simulink model "TEP_Final_NoScript"  (R2024a)
settings: Solver=FixedStepAuto  StartTime=0.0  StopTime=10  FixedStep=1/3600  RelTol=1e-3
model workspace (MAT data in the model file):
  AD : Simulink.Parameter (value not decoded)
  AG : Simulink.Parameter (value not decoded)
  AH : Simulink.Parameter (value not decoded)
  AV : Simulink.Parameter (value not decoded)
  AVP : Simulink.Parameter (value not decoded)
  BCHL : Simulink.Parameter (value not decoded)
  BCHV : Simulink.Parameter (value not decoded)
  BD : Simulink.Parameter (value not decoded)
  BG : Simulink.Parameter (value not decoded)
  BH : Simulink.Parameter (value not decoded)
  BVP : Simulink.Parameter (value not decoded)
  CD : Simulink.Parameter (value not decoded)
  CG : Simulink.Parameter (value not decoded)
  CH : Simulink.Parameter (value not decoded)
  CVP : Simulink.Parameter (value not decoded)
  XMW : Simulink.Parameter (value not decoded)
  XNS : Simulink.Parameter (value not decoded)
  XNSE : Simulink.Parameter (value not decoded)
symbols that are objects in the model workspace (value not decoded): AD, AG, AH, AV, AVP, BD, BG, BH, BVP, CD, CG, CH, CVP, XMW, XNS, XNSE
undefined symbols (not defined in the file or in its folder): magnitude, msgbox, SETPT, XMEAS, XMV
libraries: mylib x360, dspindex x28
(part 12 of 14)

== system TEP_Final_NoScript/Subsystem1/RCout/Subsystem3/Subsystem/Subsystem2 ==
  T1 : Inport
  T0 : Inport  Port=2
  A : Constant  Value=9.069
  Add1 : Sum  Inputs=+-
  Product1 : Product
  AT : Outport
  wires:
  Add1/1 -> Product1/2
  A/1 -> Product1/1
  T0/1 -> Add1/2
  T1/1 -> Add1/1
  Product1/1 -> AT/1

== system TEP_Final_NoScript/Subsystem1/RCout/Subsystem3/Subsystem1/Subsystem ==
  T1 : Inport
  T0 : Inport  Port=2
  A : Constant  Value=9.069
  Divide : Product  Inputs=*/
  Math Function : Math  Operator=log  SignedPower=on
  Product1 : Product
  AT : Outport
  wires:
  Product1/1 -> AT/1
  A/1 -> Product1/1
  T1/1 -> Divide/1
  T0/1 -> Divide/2
  Math Function/1 -> Product1/2
  Divide/1 -> Math Function/1

== system TEP_Final_NoScript/Subsystem1/Reactor feed stream/Composition measurement mol%/Subsystem/Subsystem ==
  XST : Inport
  Constant : Constant  Value=100
  Multiport Selector : dspindex/Multiport Selector  rowsOrCols=Rows  idxCellArray={7,8}  idxErrMode=Clip Index
  Product6 : Product
  Product7 : Product
  XCMPG : Outport  VectorParamsAs1DForOutWhenUnconnected=off
  "XCMPH " : Outport  Port=2  VectorParamsAs1DForOutWhenUnconnected=off
  wires:
  Multiport Selector/2 -> Product7/1
  Multiport Selector/1 -> Product6/1
  Constant/1 -> Product6/2, Product7/2
  XST/1 -> Multiport Selector/1
  Product6/1 -> XCMPG/1
  Product7/1 -> "XCMPH "/1

== system TEP_Final_NoScript/Subsystem1/Reactor product stream/Composition measurement mol%/Subsystem/Subsystem ==
  XST : Inport
  Constant : Constant  Value=100
  Multiport Selector : dspindex/Multiport Selector  rowsOrCols=Rows  idxCellArray={ 1,2,3,4,5,6,7,8}  idxErrMode=Clip Index
  Product{,1..7} (8 alike) : Product
  XCMPA : Outport  VectorParamsAs1DForOutWhenUnconnected=off
  XCMPB : Outport  Port=2  VectorParamsAs1DForOutWhenUnconnected=off
  XCMPC : Outport  Port=3  VectorParamsAs1DForOutWhenUnconnected=off
  XCMPD : Outport  Port=4  VectorParamsAs1DForOutWhenUnconnected=off
  "XCMPE " : Outport  Port=5  VectorParamsAs1DForOutWhenUnconnected=off
  "XCMPF " : Outport  Port=6  VectorParamsAs1DForOutWhenUnconnected=off
  XCMPG : Outport  Port=7  VectorParamsAs1DForOutWhenUnconnected=off
  "XCMPH " : Outport  Port=8  VectorParamsAs1DForOutWhenUnconnected=off
  wires:
  Multiport Selector/6 -> Product5/1
  Multiport Selector/8 -> Product7/1
  Multiport Selector/5 -> Product4/1
  Multiport Selector/7 -> Product6/1
  Multiport Selector/1 -> Product/1
  Multiport Selector/3 -> Product2/1
  Constant/1 -> Product/2, Product1/2, Product2/2, Product3/2, Product4/2, Product5/2, Product7/2, Product6/2
  Multiport Selector/4 -> Product3/1
  XST/1 -> Multiport Selector/1
  Multiport Selector/2 -> Product1/1
  Product/1 -> XCMPA/1
  Product1/1 -> XCMPB/1
  Product2/1 -> XCMPC/1
  Product3/1 -> XCMPD/1
  Product4/1 -> "XCMPE "/1
  Product5/1 -> "XCMPF "/1
  Product6/1 -> XCMPG/1
  Product7/1 -> "XCMPH "/1

== system TEP_Final_NoScript/Subsystem1/Separator recycle stream/Composition measurement mol%/Subsystem/Subsystem ==
  XST : Inport
  Constant : Constant  Value=100
  Multiport Selector : dspindex/Multiport Selector  rowsOrCols=Rows  idxCellArray={ 1,2,3,4,5,6,7,8}  idxErrMode=Clip Index
  Product{,1..7} (8 alike) : Product
  XCMPA : Outport  VectorParamsAs1DForOutWhenUnconnected=off
  XCMPB : Outport  Port=2  VectorParamsAs1DForOutWhenUnconnected=off
  XCMPC : Outport  Port=3  VectorParamsAs1DForOutWhenUnconnected=off
  XCMPD : Outport  Port=4  VectorParamsAs1DForOutWhenUnconnected=off
  "XCMPE " : Outport  Port=5  VectorParamsAs1DForOutWhenUnconnected=off
  "XCMPF " : Outport  Port=6  VectorParamsAs1DForOutWhenUnconnected=off
  XCMPG : Outport  Port=7  VectorParamsAs1DForOutWhenUnconnected=off
  "XCMPH " : Outport  Port=8  VectorParamsAs1DForOutWhenUnconnected=off
  wires:
  Multiport Selector/6 -> Product5/1
  Multiport Selector/8 -> Product7/1
  Multiport Selector/5 -> Product4/1
  Multiport Selector/7 -> Product6/1
  Multiport Selector/1 -> Product/1
  Multiport Selector/3 -> Product2/1
  Constant/1 -> Product/2, Product1/2, Product2/2, Product3/2, Product4/2, Product5/2, Product7/2, Product6/2
  Multiport Selector/4 -> Product3/1
  XST/1 -> Multiport Selector/1
  Multiport Selector/2 -> Product1/1
  Product/1 -> XCMPA/1
  Product1/1 -> XCMPB/1
  Product2/1 -> XCMPC/1
  Product3/1 -> XCMPD/1
  Product4/1 -> "XCMPE "/1
  Product5/1 -> "XCMPF "/1
  Product6/1 -> XCMPG/1
  Product7/1 -> "XCMPH "/1

== system TEP_Final_NoScript/Subsystem1/Separator underflow stream/Composition measurement mol%/Subsystem/Subsystem ==
  XST : Inport
  Constant : Constant  Value=100
  Multiport Selector : dspindex/Multiport Selector  rowsOrCols=Rows  idxCellArray={ 1,2,3,4,5,6,7,8}  idxErrMode=Clip Index
  Product{,1..7} (8 alike) : Product
  XCMPA : Outport  VectorParamsAs1DForOutWhenUnconnected=off
  XCMPB : Outport  Port=2  VectorParamsAs1DForOutWhenUnconnected=off
  XCMPC : Outport  Port=3  VectorParamsAs1DForOutWhenUnconnected=off
  XCMPD : Outport  Port=4  VectorParamsAs1DForOutWhenUnconnected=off
  "XCMPE " : Outport  Port=5  VectorParamsAs1DForOutWhenUnconnected=off
  "XCMPF " : Outport  Port=6  VectorParamsAs1DForOutWhenUnconnected=off
  XCMPG : Outport  Port=7  VectorParamsAs1DForOutWhenUnconnected=off
  "XCMPH " : Outport  Port=8  VectorParamsAs1DForOutWhenUnconnected=off
  wires:
  Multiport Selector/6 -> Product5/1
  Multiport Selector/8 -> Product7/1
  Multiport Selector/5 -> Product4/1
  Multiport Selector/7 -> Product6/1
  Multiport Selector/1 -> Product/1
  Multiport Selector/3 -> Product2/1
  Constant/1 -> Product/2, Product1/2, Product2/2, Product3/2, Product4/2, Product5/2, Product7/2, Product6/2
  Multiport Selector/4 -> Product3/1
  XST/1 -> Multiport Selector/1
  Multiport Selector/2 -> Product1/1
  Product/1 -> XCMPA/1
  Product1/1 -> XCMPB/1
  Product2/1 -> XCMPC/1
  Product3/1 -> XCMPD/1
  Product4/1 -> "XCMPE "/1
  Product5/1 -> "XCMPF "/1
  Product6/1 -> XCMPG/1
  Product7/1 -> "XCMPH "/1

== system TEP_Final_NoScript/Subsystem1/Stripper recycle stream/Composition measurement mol%/Subsystem/Subsystem ==
  XST : Inport
  Constant : Constant  Value=100
  Multiport Selector : dspindex/Multiport Selector  rowsOrCols=Rows  idxCellArray={ 1,2,3,4,5,6,7,8}  idxErrMode=Clip Index
  Product{,1..7} (8 alike) : Product
  XCMPA : Outport  VectorParamsAs1DForOutWhenUnconnected=off
  XCMPB : Outport  Port=2  VectorParamsAs1DForOutWhenUnconnected=off
  XCMPC : Outport  Port=3  VectorParamsAs1DForOutWhenUnconnected=off
  XCMPD : Outport  Port=4  VectorParamsAs1DForOutWhenUnconnected=off
  "XCMPE " : Outport  Port=5  VectorParamsAs1DForOutWhenUnconnected=off
  "XCMPF " : Outport  Port=6  VectorParamsAs1DForOutWhenUnconnected=off
  XCMPG : Outport  Port=7  VectorParamsAs1DForOutWhenUnconnected=off
  "XCMPH " : Outport  Port=8  VectorParamsAs1DForOutWhenUnconnected=off
  wires:
  Multiport Selector/6 -> Product5/1
  Multiport Selector/8 -> Product7/1
  Multiport Selector/5 -> Product4/1
  Multiport Selector/7 -> Product6/1
  Multiport Selector/1 -> Product/1
  Multiport Selector/3 -> Product2/1
  Constant/1 -> Product/2, Product1/2, Product2/2, Product3/2, Product4/2, Product5/2, Product7/2, Product6/2
  Multiport Selector/4 -> Product3/1
  XST/1 -> Multiport Selector/1
  Multiport Selector/2 -> Product1/1
  Product/1 -> XCMPA/1
  Product1/1 -> XCMPB/1
  Product2/1 -> XCMPC/1
  Product3/1 -> XCMPD/1
  Product4/1 -> "XCMPE "/1
  Product5/1 -> "XCMPF "/1
  Product6/1 -> XCMPG/1
  Product7/1 -> "XCMPH "/1

== system TEP_Final_NoScript/Subsystem1/Subsystem1/Subsystem1/Flow measurement in lb-mol//hr/XMWS Molecular weight of Stream lb//lb-mol ==
  XST : Inport
  Product : Product
  Sum of Elements : Sum  Inputs=+
  "XMW(I) Molecular weight of components lb/lb-mol " : Constant  Value=XMW
  XMWS : Outport  VectorParamsAs1DForOutWhenUnconnected=off
  wires:
  Sum of Elements/1 -> XMWS/1
  Product/1 -> Sum of Elements/1
  XST/1 -> Product/1
  "XMW(I) Molecular weight of components lb/lb-mol "/1 -> Product/2

== system TEP_Final_NoScript/Subsystem1/Subsystem13/Subsystem1/Flow measurement in lb-mol//hr/XMWS Molecular weight of Stream lb//lb-mol ==
  XST : Inport
  Product : Product
  Sum of Elements : Sum  Inputs=+
  "XMW(I) Molecular weight of components lb/lb-mol " : Constant  Value=XMW
  XMWS : Outport  VectorParamsAs1DForOutWhenUnconnected=off
  wires:
  Sum of Elements/1 -> XMWS/1
  Product/1 -> Sum of Elements/1
  XST/1 -> Product/1
  "XMW(I) Molecular weight of components lb/lb-mol "/1 -> Product/2

== system TEP_Final_NoScript/Subsystem1/Subsystem14/Subsystem1/Flow measurement in lb-mol//hr/XMWS Molecular weight of Stream lb//lb-mol ==
  XST : Inport
  Product : Product
  Sum of Elements : Sum  Inputs=+
  "XMW(I) Molecular weight of components lb/lb-mol " : Constant  Value=XMW
  XMWS : Outport  VectorParamsAs1DForOutWhenUnconnected=off
  wires:
  Sum of Elements/1 -> XMWS/1
  Product/1 -> Sum of Elements/1
  XST/1 -> Product/1
  "XMW(I) Molecular weight of components lb/lb-mol "/1 -> Product/2

== system TEP_Final_NoScript/Subsystem1/Subsystem15/Subsystem1/Flow measurement in lb-mol//hr/XMWS Molecular weight of Stream lb//lb-mol ==
  XST : Inport
  Product : Product
  Sum of Elements : Sum  Inputs=+
  "XMW(I) Molecular weight of components lb/lb-mol " : Constant  Value=XMW
  XMWS : Outport  VectorParamsAs1DForOutWhenUnconnected=off
  wires:
  Sum of Elements/1 -> XMWS/1
  Product/1 -> Sum of Elements/1
  XST/1 -> Product/1
  "XMW(I) Molecular weight of components lb/lb-mol "/1 -> Product/2

== system TEP_Final_NoScript/Subsystem1/Subsystem16/Subsystem1/Flow measurement in lb-mol//hr/XMWS Molecular weight of Stream lb//lb-mol ==
  XST : Inport
  Product : Product
  Sum of Elements : Sum  Inputs=+
  "XMW(I) Molecular weight of components lb/lb-mol " : Constant  Value=XMW
  XMWS : Outport  VectorParamsAs1DForOutWhenUnconnected=off
  wires:
  Sum of Elements/1 -> XMWS/1
  Product/1 -> Sum of Elements/1
  XST/1 -> Product/1
  "XMW(I) Molecular weight of components lb/lb-mol "/1 -> Product/2

== system TEP_Final_NoScript/Subsystem1/Subsystem17/Subsystem1/Flow measurement in lb-mol//hr/XMWS Molecular weight of Stream lb//lb-mol ==
  XST : Inport
  Product : Product
  Sum of Elements : Sum  Inputs=+
  "XMW(I) Molecular weight of components lb/lb-mol " : Constant  Value=XMW
  XMWS : Outport  VectorParamsAs1DForOutWhenUnconnected=off
  wires:
  Sum of Elements/1 -> XMWS/1
  Product/1 -> Sum of Elements/1
  XST/1 -> Product/1
  "XMW(I) Molecular weight of components lb/lb-mol "/1 -> Product/2

== system TEP_Final_NoScript/Subsystem1/Subsystem2/Subsystem1/Flow measurement in lb-mol//hr/XMWS Molecular weight of Stream lb//lb-mol ==
  XST : Inport
  Product : Product
  Sum of Elements : Sum  Inputs=+
  "XMW(I) Molecular weight of components lb/lb-mol " : Constant  Value=XMW
  XMWS : Outport  VectorParamsAs1DForOutWhenUnconnected=off
  wires:
  Sum of Elements/1 -> XMWS/1
  Product/1 -> Sum of Elements/1
  XST/1 -> Product/1
  "XMW(I) Molecular weight of components lb/lb-mol "/1 -> Product/2

== system TEP_Final_NoScript/Subsystem1/Subsystem3/Subsystem1/Flow measurement in lb-mol//hr/XMWS Molecular weight of Stream lb//lb-mol ==
  XST : Inport
  Product : Product
  Sum of Elements : Sum  Inputs=+
  "XMW(I) Molecular weight of components lb/lb-mol " : Constant  Value=XMW
  XMWS : Outport  VectorParamsAs1DForOutWhenUnconnected=off
  wires:
  Sum of Elements/1 -> XMWS/1
  Product/1 -> Sum of Elements/1
  XST/1 -> Product/1
  "XMW(I) Molecular weight of components lb/lb-mol "/1 -> Product/2

== system TEP_Final_NoScript/Subsystem1/Subsystem4/Subsystem1/Flow measurement in lb-mol//hr/XMWS Molecular weight of Stream lb//lb-mol ==
  XST : Inport
  Product : Product
  Sum of Elements : Sum  Inputs=+
  "XMW(I) Molecular weight of components lb/lb-mol " : Constant  Value=XMW
  XMWS : Outport  VectorParamsAs1DForOutWhenUnconnected=off
  wires:
  Sum of Elements/1 -> XMWS/1
  Product/1 -> Sum of Elements/1
  XST/1 -> Product/1
  "XMW(I) Molecular weight of components lb/lb-mol "/1 -> Product/2

== system TEP_Final_NoScript/Subsystem1/Subsystem5/Subsystem1/Flow measurement in lb-mol//hr/XMWS Molecular weight of Stream lb//lb-mol ==
  XST : Inport
  Product : Product
  Sum of Elements : Sum  Inputs=+
  "XMW(I) Molecular weight of components lb/lb-mol " : Constant  Value=XMW
  XMWS : Outport  VectorParamsAs1DForOutWhenUnconnected=off
  wires:
  Sum of Elements/1 -> XMWS/1
  Product/1 -> Sum of Elements/1
  XST/1 -> Product/1
  "XMW(I) Molecular weight of components lb/lb-mol "/1 -> Product/2

== system TEP_Final_NoScript/Subsystem1/Subsystem8/Subsystem1/Flow measurement in lb-mol//hr/XMWS Molecular weight of Stream lb//lb-mol ==
  XST : Inport
  Product : Product
  Sum of Elements : Sum  Inputs=+
  "XMW(I) Molecular weight of components lb/lb-mol " : Constant  Value=XMW
  XMWS : Outport  VectorParamsAs1DForOutWhenUnconnected=off
  wires:
  Sum of Elements/1 -> XMWS/1
  Product/1 -> Sum of Elements/1
  XST/1 -> Product/1
  "XMW(I) Molecular weight of components lb/lb-mol "/1 -> Product/2

== system TEP_Final_NoScript/Random number generator1/Process Measurements XMEAS(I) I=23-36/If Action Subsystem3/Subsystem/Subsystem/TESUB6 XMNS(23) ==
  G : Inport
  Process Noise I=1-12 G New : mylib/Process Noise I=1-12 G New  SystemSampleTime=-1  VariantActivationTime=update diagram  AllowFlexibleInterface=on  Latency=0  AutoFrameSizeCalculation=off
      settings: SourceProductName=TEP Library
  XNS(23) : Constant  Value=0.25
  XMNS : Outport  VectorParamsAs1DForOutWhenUnconnected=off
  G_NEW : Outport  Port=2  VectorParamsAs1DForOutWhenUnconnected=off
  wires:
  XNS(23)/1 -> Process Noise I=1-12 G New/1
  Process Noise I=1-12 G New/1 -> XMNS/1
  G/1 -> Process Noise I=1-12 G New/2
  Process Noise I=1-12 G New/2 -> G_NEW/1

== system TEP_Final_NoScript/Random number generator1/Process Measurements XMEAS(I) I=23-36/If Action Subsystem3/Subsystem/Subsystem/TESUB6 XMNS(24) ==
  G : Inport
  Process Noise I=1-12 G New : mylib/Process Noise I=1-12 G New  SystemSampleTime=-1  VariantActivationTime=update diagram  AllowFlexibleInterface=on  Latency=0  AutoFrameSizeCalculation=off
      settings: SourceProductName=TEP Library
  XNS(24) : Constant  Value=0.1
  XMNS : Outport  VectorParamsAs1DForOutWhenUnconnected=off
  G_NEW : Outport  Port=2  VectorParamsAs1DForOutWhenUnconnected=off
  wires:
  XNS(24)/1 -> Process Noise I=1-12 G New/1
  Process Noise I=1-12 G New/1 -> XMNS/1
  G/1 -> Process Noise I=1-12 G New/2
  Process Noise I=1-12 G New/2 -> G_NEW/1

== system TEP_Final_NoScript/Random number generator1/Process Measurements XMEAS(I) I=23-36/If Action Subsystem3/Subsystem/Subsystem/TESUB6 XMNS(25) ==
  G : Inport
  Process Noise I=1-12 G New : mylib/Process Noise I=1-12 G New  SystemSampleTime=-1  VariantActivationTime=update diagram  AllowFlexibleInterface=on  Latency=0  AutoFrameSizeCalculation=off
      settings: SourceProductName=TEP Library
  XNS(25) : Constant  Value=0.25
  XMNS : Outport  VectorParamsAs1DForOutWhenUnconnected=off
  G_NEW : Outport  Port=2  VectorParamsAs1DForOutWhenUnconnected=off
  wires:
  XNS(25)/1 -> Process Noise I=1-12 G New/1
  Process Noise I=1-12 G New/1 -> XMNS/1
  G/1 -> Process Noise I=1-12 G New/2
  Process Noise I=1-12 G New/2 -> G_NEW/1

== system TEP_Final_NoScript/Random number generator1/Process Measurements XMEAS(I) I=23-36/If Action Subsystem3/Subsystem/Subsystem/TESUB6 XMNS(26) ==
  G : Inport
  Process Noise I=1-12 G New : mylib/Process Noise I=1-12 G New  SystemSampleTime=-1  VariantActivationTime=update diagram  AllowFlexibleInterface=on  Latency=0  AutoFrameSizeCalculation=off
      settings: SourceProductName=TEP Library
  XNS(26) : Constant  Value=0.1
  XMNS : Outport  VectorParamsAs1DForOutWhenUnconnected=off
  G_NEW : Outport  Port=2  VectorParamsAs1DForOutWhenUnconnected=off
  wires:
  XNS(26)/1 -> Process Noise I=1-12 G New/1
  Process Noise I=1-12 G New/1 -> XMNS/1
  G/1 -> Process Noise I=1-12 G New/2
  Process Noise I=1-12 G New/2 -> G_NEW/1

== system TEP_Final_NoScript/Random number generator1/Process Measurements XMEAS(I) I=23-36/If Action Subsystem3/Subsystem/Subsystem/TESUB6 XMNS(27) ==
  G : Inport
  Process Noise I=1-12 G New : mylib/Process Noise I=1-12 G New  SystemSampleTime=-1  VariantActivationTime=update diagram  AllowFlexibleInterface=on  Latency=0  AutoFrameSizeCalculation=off
      settings: SourceProductName=TEP Library
  XNS(27) : Constant  Value=0.25
  XMNS : Outport  VectorParamsAs1DForOutWhenUnconnected=off
  G_NEW : Outport  Port=2  VectorParamsAs1DForOutWhenUnconnected=off
  wires:
  XNS(27)/1 -> Process Noise I=1-12 G New/1
  Process Noise I=1-12 G New/1 -> XMNS/1
  G/1 -> Process Noise I=1-12 G New/2
  Process Noise I=1-12 G New/2 -> G_NEW/1

== system TEP_Final_NoScript/Random number generator1/Process Measurements XMEAS(I) I=23-36/If Action Subsystem3/Subsystem/Subsystem1/TESUB6 XMNS(28) ==
  G : Inport
  Process Noise I=1-12 G New : mylib/Process Noise I=1-12 G New  SystemSampleTime=-1  VariantActivationTime=update diagram  AllowFlexibleInterface=on  Latency=0  AutoFrameSizeCalculation=off
      settings: SourceProductName=TEP Library
  XNS(28) : Constant  Value=0.025
  XMNS : Outport  VectorParamsAs1DForOutWhenUnconnected=off
  G_NEW : Outport  Port=2  VectorParamsAs1DForOutWhenUnconnected=off
  wires:
  XNS(28)/1 -> Process Noise I=1-12 G New/1
  Process Noise I=1-12 G New/1 -> XMNS/1
  G/1 -> Process Noise I=1-12 G New/2
  Process Noise I=1-12 G New/2 -> G_NEW/1

== system TEP_Final_NoScript/Random number generator1/Process Measurements XMEAS(I) I=23-36/If Action Subsystem3/Subsystem/Subsystem1/TESUB6 XMNS(29) ==
  G : Inport
  Process Noise I=1-12 G New : mylib/Process Noise I=1-12 G New  SystemSampleTime=-1  VariantActivationTime=update diagram  AllowFlexibleInterface=on  Latency=0  AutoFrameSizeCalculation=off
      settings: SourceProductName=TEP Library
  XNS(29) : Constant  Value=0.25
  XMNS : Outport  VectorParamsAs1DForOutWhenUnconnected=off
  G_NEW : Outport  Port=2  VectorParamsAs1DForOutWhenUnconnected=off
  wires:
  XNS(29)/1 -> Process Noise I=1-12 G New/1
  Process Noise I=1-12 G New/1 -> XMNS/1
  G/1 -> Process Noise I=1-12 G New/2
  Process Noise I=1-12 G New/2 -> G_NEW/1

== system TEP_Final_NoScript/Random number generator1/Process Measurements XMEAS(I) I=23-36/If Action Subsystem3/Subsystem/Subsystem1/TESUB6 XMNS(30) ==
  G : Inport
  Process Noise I=1-12 G New : mylib/Process Noise I=1-12 G New  SystemSampleTime=-1  VariantActivationTime=update diagram  AllowFlexibleInterface=on  Latency=0  AutoFrameSizeCalculation=off
      settings: SourceProductName=TEP Library
  XNS(30) : Constant  Value=0.1
  XMNS : Outport  VectorParamsAs1DForOutWhenUnconnected=off
  G_NEW : Outport  Port=2  VectorParamsAs1DForOutWhenUnconnected=off
  wires:
  XNS(30)/1 -> Process Noise I=1-12 G New/1
  Process Noise I=1-12 G New/1 -> XMNS/1
  G/1 -> Process Noise I=1-12 G New/2
  Process Noise I=1-12 G New/2 -> G_NEW/1

== system TEP_Final_NoScript/Random number generator1/Process Measurements XMEAS(I) I=23-36/If Action Subsystem3/Subsystem/Subsystem1/TESUB6 XMNS(31) ==
  G : Inport
  Process Noise I=1-12 G New : mylib/Process Noise I=1-12 G New  SystemSampleTime=-1  VariantActivationTime=update diagram  AllowFlexibleInterface=on  Latency=0  AutoFrameSizeCalculation=off
      settings: SourceProductName=TEP Library
  XNS(31) : Constant  Value=0.25
  XMNS : Outport  VectorParamsAs1DForOutWhenUnconnected=off
  G_NEW : Outport  Port=2  VectorParamsAs1DForOutWhenUnconnected=off
  wires:
  XNS(31)/1 -> Process Noise I=1-12 G New/1
  Process Noise I=1-12 G New/1 -> XMNS/1
  G/1 -> Process Noise I=1-12 G New/2
  Process Noise I=1-12 G New/2 -> G_NEW/1

== system TEP_Final_NoScript/Random number generator1/Process Measurements XMEAS(I) I=23-36/If Action Subsystem3/Subsystem/Subsystem1/TESUB6 XMNS(32) ==
  G : Inport
  Process Noise I=1-12 G New : mylib/Process Noise I=1-12 G New  SystemSampleTime=-1  VariantActivationTime=update diagram  AllowFlexibleInterface=on  Latency=0  AutoFrameSizeCalculation=off
      settings: SourceProductName=TEP Library
  XNS(32) : Constant  Value=0.1
  XMNS : Outport  VectorParamsAs1DForOutWhenUnconnected=off
  G_NEW : Outport  Port=2  VectorParamsAs1DForOutWhenUnconnected=off
  wires:
  XNS(32)/1 -> Process Noise I=1-12 G New/1
  Process Noise I=1-12 G New/1 -> XMNS/1
  G/1 -> Process Noise I=1-12 G New/2
  Process Noise I=1-12 G New/2 -> G_NEW/1

== system TEP_Final_NoScript/Random number generator1/Process Measurements XMEAS(I) I=23-36/If Action Subsystem3/Subsystem/Subsystem2/TESUB6 XMNS(33) ==
  G : Inport
  Process Noise I=1-12 G New : mylib/Process Noise I=1-12 G New  SystemSampleTime=-1  VariantActivationTime=update diagram  AllowFlexibleInterface=on  Latency=0  AutoFrameSizeCalculation=off
      settings: SourceProductName=TEP Library
  XNS(33) : Constant  Value=0.25
  XMNS : Outport  VectorParamsAs1DForOutWhenUnconnected=off
  G_NEW : Outport  Port=2  VectorParamsAs1DForOutWhenUnconnected=off
  wires:
  XNS(33)/1 -> Process Noise I=1-12 G New/1
  Process Noise I=1-12 G New/1 -> XMNS/1
  G/1 -> Process Noise I=1-12 G New/2
  Process Noise I=1-12 G New/2 -> G_NEW/1

== system TEP_Final_NoScript/Random number generator1/Process Measurements XMEAS(I) I=23-36/If Action Subsystem3/Subsystem/Subsystem2/TESUB6 XMNS(34) ==
  G : Inport
  Process Noise I=1-12 G New : mylib/Process Noise I=1-12 G New  SystemSampleTime=-1  VariantActivationTime=update diagram  AllowFlexibleInterface=on  Latency=0  AutoFrameSizeCalculation=off
      settings: SourceProductName=TEP Library
  XNS(34) : Constant  Value=0.025
  XMNS : Outport  VectorParamsAs1DForOutWhenUnconnected=off
  G_NEW : Outport  Port=2  VectorParamsAs1DForOutWhenUnconnected=off
  wires:
  XNS(34)/1 -> Process Noise I=1-12 G New/1
  Process Noise I=1-12 G New/1 -> XMNS/1
  G/1 -> Process Noise I=1-12 G New/2
  Process Noise I=1-12 G New/2 -> G_NEW/1

== system TEP_Final_NoScript/Random number generator1/Process Measurements XMEAS(I) I=23-36/If Action Subsystem3/Subsystem/Subsystem2/TESUB6 XMNS(35) ==
  G : Inport
  Process Noise I=1-12 G New : mylib/Process Noise I=1-12 G New  SystemSampleTime=-1  VariantActivationTime=update diagram  AllowFlexibleInterface=on  Latency=0  AutoFrameSizeCalculation=off
      settings: SourceProductName=TEP Library
  XNS(35) : Constant  Value=0.05
  XMNS : Outport  VectorParamsAs1DForOutWhenUnconnected=off
  G_NEW : Outport  Port=2  VectorParamsAs1DForOutWhenUnconnected=off
  wires:
  XNS(35)/1 -> Process Noise I=1-12 G New/1
  Process Noise I=1-12 G New/1 -> XMNS/1
  G/1 -> Process Noise I=1-12 G New/2
  Process Noise I=1-12 G New/2 -> G_NEW/1

== system TEP_Final_NoScript/Random number generator1/Process Measurements XMEAS(I) I=23-36/If Action Subsystem3/Subsystem/Subsystem2/TESUB6 XMNS(36) ==
  G : Inport
  Process Noise I=1-12 G New : mylib/Process Noise I=1-12 G New  SystemSampleTime=-1  VariantActivationTime=update diagram  AllowFlexibleInterface=on  Latency=0  AutoFrameSizeCalculation=off
      settings: SourceProductName=TEP Library
  XNS(36) : Constant  Value=0.05
  XMNS : Outport  VectorParamsAs1DForOutWhenUnconnected=off
  G_NEW : Outport  Port=2  VectorParamsAs1DForOutWhenUnconnected=off
  wires:
  XNS(36)/1 -> Process Noise I=1-12 G New/1
  Process Noise I=1-12 G New/1 -> XMNS/1
  G/1 -> Process Noise I=1-12 G New/2
  Process Noise I=1-12 G New/2 -> G_NEW/1

== system TEP_Final_NoScript/Random number generator1/Process Measurements XMEAS(I) I=37-41/If Action Subsystem3/Subsystem/Subsystem/TESUB6 XMNS(37) ==
  G : Inport
  Process Noise I=1-12 G New : mylib/Process Noise I=1-12 G New  SystemSampleTime=-1  VariantActivationTime=update diagram  AllowFlexibleInterface=on  Latency=0  AutoFrameSizeCalculation=off
      settings: SourceProductName=TEP Library
  XNS(37) : Constant  Value=0.01
  XMNS : Outport  VectorParamsAs1DForOutWhenUnconnected=off
  G_NEW : Outport  Port=2  VectorParamsAs1DForOutWhenUnconnected=off
  wires:
  XNS(37)/1 -> Process Noise I=1-12 G New/1
  Process Noise I=1-12 G New/1 -> XMNS/1
  G/1 -> Process Noise I=1-12 G New/2
  Process Noise I=1-12 G New/2 -> G_NEW/1

== system TEP_Final_NoScript/Random number generator1/Process Measurements XMEAS(I) I=37-41/If Action Subsystem3/Subsystem/Subsystem/TESUB6 XMNS(38) ==
  G : Inport
  Process Noise I=1-12 G New : mylib/Process Noise I=1-12 G New  SystemSampleTime=-1  VariantActivationTime=update diagram  AllowFlexibleInterface=on  Latency=0  AutoFrameSizeCalculation=off
      settings: SourceProductName=TEP Library
  XNS(38) : Constant  Value=0.01
  XMNS : Outport  VectorParamsAs1DForOutWhenUnconnected=off
  G_NEW : Outport  Port=2  VectorParamsAs1DForOutWhenUnconnected=off
  wires:
  XNS(38)/1 -> Process Noise I=1-12 G New/1
  Process Noise I=1-12 G New/1 -> XMNS/1
  G/1 -> Process Noise I=1-12 G New/2
  Process Noise I=1-12 G New/2 -> G_NEW/1

== system TEP_Final_NoScript/Random number generator1/Process Measurements XMEAS(I) I=37-41/If Action Subsystem3/Subsystem/Subsystem/TESUB6 XMNS(39) ==
  G : Inport
  Process Noise I=1-12 G New : mylib/Process Noise I=1-12 G New  SystemSampleTime=-1  VariantActivationTime=update diagram  AllowFlexibleInterface=on  Latency=0  AutoFrameSizeCalculation=off
      settings: SourceProductName=TEP Library
  XNS(39) : Constant  Value=0.01
  XMNS : Outport  VectorParamsAs1DForOutWhenUnconnected=off
  G_NEW : Outport  Port=2  VectorParamsAs1DForOutWhenUnconnected=off
  wires:
  XNS(39)/1 -> Process Noise I=1-12 G New/1
  Process Noise I=1-12 G New/1 -> XMNS/1
  G/1 -> Process Noise I=1-12 G New/2
  Process Noise I=1-12 G New/2 -> G_NEW/1

== system TEP_Final_NoScript/Random number generator1/Process Measurements XMEAS(I) I=37-41/If Action Subsystem3/Subsystem/Subsystem/TESUB6 XMNS(40) ==
  G : Inport
  Process Noise I=1-12 G New : mylib/Process Noise I=1-12 G New  SystemSampleTime=-1  VariantActivationTime=update diagram  AllowFlexibleInterface=on  Latency=0  AutoFrameSizeCalculation=off
      settings: SourceProductName=TEP Library
  XNS(40) : Constant  Value=0.5
  XMNS : Outport  VectorParamsAs1DForOutWhenUnconnected=off
  G_NEW : Outport  Port=2  VectorParamsAs1DForOutWhenUnconnected=off
  wires:
  XNS(40)/1 -> Process Noise I=1-12 G New/1
  Process Noise I=1-12 G New/1 -> XMNS/1
  G/1 -> Process Noise I=1-12 G New/2
  Process Noise I=1-12 G New/2 -> G_NEW/1

== system TEP_Final_NoScript/Random number generator1/Process Measurements XMEAS(I) I=37-41/If Action Subsystem3/Subsystem/Subsystem/TESUB6 XMNS(41) ==
  G : Inport
  Process Noise I=1-12 G New : mylib/Process Noise I=1-12 G New  SystemSampleTime=-1  VariantActivationTime=update diagram  AllowFlexibleInterface=on  Latency=0  AutoFrameSizeCalculation=off
      settings: SourceProductName=TEP Library
  XNS(41) : Constant  Value=0.5
  XMNS : Outport  VectorParamsAs1DForOutWhenUnconnected=off
  G_NEW : Outport  Port=2  VectorParamsAs1DForOutWhenUnconnected=off
  wires:
  XNS(41)/1 -> Process Noise I=1-12 G New/1
  Process Noise I=1-12 G New/1 -> XMNS/1
  G/1 -> Process Noise I=1-12 G New/2
  Process Noise I=1-12 G New/2 -> G_NEW/1

== system TEP_Final_NoScript/Random number generator1/Stream Measurements SMEAS Gas analysis/If Action Subsystem3/Subsystem/Stream 1/Subsystem ==
  G : Inport
  TESUB6 XMNSEA : Subsystem
  TESUB6 XMNSEB : Subsystem
  TESUB6 XMNSEC : Subsystem
  TESUB6 XMNSED : Subsystem
  TESUB6 XMNSEE : Subsystem
  TESUB6 XMNSEF : Subsystem
  TESUB6 XMNSEG : Subsystem
  TESUB6 XMNSEH : Subsystem
  XMNSEA : Outport  VectorParamsAs1DForOutWhenUnconnected=off
  XMNSEB : Outport  Port=2  VectorParamsAs1DForOutWhenUnconnected=off
  XMNSEC : Outport  Port=3  VectorParamsAs1DForOutWhenUnconnected=off
  XMNSED : Outport  Port=4  VectorParamsAs1DForOutWhenUnconnected=off
  XMNSEE : Outport  Port=5  VectorParamsAs1DForOutWhenUnconnected=off
  XMNSEF : Outport  Port=6  VectorParamsAs1DForOutWhenUnconnected=off
  XMNSEG : Outport  Port=7  VectorParamsAs1DForOutWhenUnconnected=off
  XMNSEH : Outport  Port=8  VectorParamsAs1DForOutWhenUnconnected=off
  G_NEW : Outport  Port=9  VectorParamsAs1DForOutWhenUnconnected=off
  wires:
  TESUB6 XMNSEB/2(G_NEW) -> TESUB6 XMNSEC/1(G)
  G/1 -> TESUB6 XMNSEA/1(G)
  TESUB6 XMNSEA/2(G_NEW) -> TESUB6 XMNSEB/1(G)
  TESUB6 XMNSEC/2(G_NEW) -> TESUB6 XMNSED/1(G)
  TESUB6 XMNSED/1(XMNSED) -> XMNSED/1  "XMNSED"
  TESUB6 XMNSEE/1(XMNSEE) -> XMNSEE/1  "XMNSEE"
  TESUB6 XMNSED/2(G_NEW) -> TESUB6 XMNSEE/1(G)
  TESUB6 XMNSEC/1(XMNSEC) -> XMNSEC/1  "XMNSEC"
  TESUB6 XMNSEA/1(XMNSEA) -> XMNSEA/1  "XMNSEA"
  TESUB6 XMNSEB/1(XMNSEB) -> XMNSEB/1  "XMNSEB"
  TESUB6 XMNSEE/2(G_NEW) -> TESUB6 XMNSEF/1(G)
  TESUB6 XMNSEF/2(G_NEW) -> TESUB6 XMNSEG/1(G)
  TESUB6 XMNSEG/2(G_NEW) -> TESUB6 XMNSEH/1(G)
  TESUB6 XMNSEH/2(G_NEW) -> G_NEW/1
  TESUB6 XMNSEF/1(XMNSEF) -> XMNSEF/1  "XMNSEF"
  TESUB6 XMNSEG/1(XMNSEG) -> XMNSEG/1  "XMNSEG"
  TESUB6 XMNSEH/1(XMNSEH) -> XMNSEH/1  "XMNSEH"

== system TEP_Final_NoScript/Random number generator1/Stream Measurements SMEAS Gas analysis/If Action Subsystem3/Subsystem/Stream 13/Subsystem ==
  G : Inport
  TESUB6 XMNSEA : Subsystem
  TESUB6 XMNSEB : Subsystem
  TESUB6 XMNSEC : Subsystem
  TESUB6 XMNSED : Subsystem
  TESUB6 XMNSEE : Subsystem
  TESUB6 XMNSEF : Subsystem
  TESUB6 XMNSEG : Subsystem
  TESUB6 XMNSEH : Subsystem
  XMNSEA : Outport  VectorParamsAs1DForOutWhenUnconnected=off
  XMNSEB : Outport  Port=2  VectorParamsAs1DForOutWhenUnconnected=off
  XMNSEC : Outport  Port=3  VectorParamsAs1DForOutWhenUnconnected=off
  XMNSED : Outport  Port=4  VectorParamsAs1DForOutWhenUnconnected=off
  XMNSEE : Outport  Port=5  VectorParamsAs1DForOutWhenUnconnected=off
  XMNSEF : Outport  Port=6  VectorParamsAs1DForOutWhenUnconnected=off
  XMNSEG : Outport  Port=7  VectorParamsAs1DForOutWhenUnconnected=off
  XMNSEH : Outport  Port=8  VectorParamsAs1DForOutWhenUnconnected=off
  G_NEW : Outport  Port=9  VectorParamsAs1DForOutWhenUnconnected=off
  wires:
  TESUB6 XMNSEB/2(G_NEW) -> TESUB6 XMNSEC/1(G)
  G/1 -> TESUB6 XMNSEA/1(G)
  TESUB6 XMNSEA/2(G_NEW) -> TESUB6 XMNSEB/1(G)
  TESUB6 XMNSEC/2(G_NEW) -> TESUB6 XMNSED/1(G)
  TESUB6 XMNSED/1(XMNSED) -> XMNSED/1  "XMNSED"
  TESUB6 XMNSEE/1(XMNSEE) -> XMNSEE/1  "XMNSEE"
  TESUB6 XMNSED/2(G_NEW) -> TESUB6 XMNSEE/1(G)
  TESUB6 XMNSEC/1(XMNSEC) -> XMNSEC/1  "XMNSEC"
  TESUB6 XMNSEA/1(XMNSEA) -> XMNSEA/1  "XMNSEA"
  TESUB6 XMNSEB/1(XMNSEB) -> XMNSEB/1  "XMNSEB"
  TESUB6 XMNSEE/2(G_NEW) -> TESUB6 XMNSEF/1(G)
  TESUB6 XMNSEF/2(G_NEW) -> TESUB6 XMNSEG/1(G)
  TESUB6 XMNSEG/2(G_NEW) -> TESUB6 XMNSEH/1(G)
  TESUB6 XMNSEH/2(G_NEW) -> G_NEW/1
  TESUB6 XMNSEF/1(XMNSEF) -> XMNSEF/1  "XMNSEF"
  TESUB6 XMNSEG/1(XMNSEG) -> XMNSEG/1  "XMNSEG"
  TESUB6 XMNSEH/1(XMNSEH) -> XMNSEH/1  "XMNSEH"

== system TEP_Final_NoScript/Random number generator1/Stream Measurements SMEAS Gas analysis/If Action Subsystem3/Subsystem/Stream 2/Subsystem ==
  G : Inport
  TESUB6 XMNSEA : Subsystem
  TESUB6 XMNSEB : Subsystem
  TESUB6 XMNSEC : Subsystem
  TESUB6 XMNSED : Subsystem
  TESUB6 XMNSEE : Subsystem
  TESUB6 XMNSEF : Subsystem
  TESUB6 XMNSEG : Subsystem
  TESUB6 XMNSEH : Subsystem
  XMNSEA : Outport  VectorParamsAs1DForOutWhenUnconnected=off
  XMNSEB : Outport  Port=2  VectorParamsAs1DForOutWhenUnconnected=off
  XMNSEC : Outport  Port=3  VectorParamsAs1DForOutWhenUnconnected=off
  XMNSED : Outport  Port=4  VectorParamsAs1DForOutWhenUnconnected=off
  XMNSEE : Outport  Port=5  VectorParamsAs1DForOutWhenUnconnected=off
  XMNSEF : Outport  Port=6  VectorParamsAs1DForOutWhenUnconnected=off
  XMNSEG : Outport  Port=7  VectorParamsAs1DForOutWhenUnconnected=off
  XMNSEH : Outport  Port=8  VectorParamsAs1DForOutWhenUnconnected=off
  G_NEW : Outport  Port=9  VectorParamsAs1DForOutWhenUnconnected=off
  wires:
  TESUB6 XMNSEB/2(G_NEW) -> TESUB6 XMNSEC/1(G)
  G/1 -> TESUB6 XMNSEA/1(G)
  TESUB6 XMNSEA/2(G_NEW) -> TESUB6 XMNSEB/1(G)
  TESUB6 XMNSEC/2(G_NEW) -> TESUB6 XMNSED/1(G)
  TESUB6 XMNSED/1(XMNSED) -> XMNSED/1  "XMNSED"
  TESUB6 XMNSEE/1(XMNSEE) -> XMNSEE/1  "XMNSEE"
  TESUB6 XMNSED/2(G_NEW) -> TESUB6 XMNSEE/1(G)
  TESUB6 XMNSEC/1(XMNSEC) -> XMNSEC/1  "XMNSEC"
  TESUB6 XMNSEA/1(XMNSEA) -> XMNSEA/1  "XMNSEA"
  TESUB6 XMNSEB/1(XMNSEB) -> XMNSEB/1  "XMNSEB"
  TESUB6 XMNSEE/2(G_NEW) -> TESUB6 XMNSEF/1(G)
  TESUB6 XMNSEF/2(G_NEW) -> TESUB6 XMNSEG/1(G)
  TESUB6 XMNSEG/2(G_NEW) -> TESUB6 XMNSEH/1(G)
  TESUB6 XMNSEH/2(G_NEW) -> G_NEW/1
  TESUB6 XMNSEF/1(XMNSEF) -> XMNSEF/1  "XMNSEF"
  TESUB6 XMNSEG/1(XMNSEG) -> XMNSEG/1  "XMNSEG"
  TESUB6 XMNSEH/1(XMNSEH) -> XMNSEH/1  "XMNSEH"

== system TEP_Final_NoScript/Random number generator1/Stream Measurements SMEAS Gas analysis/If Action Subsystem3/Subsystem/Stream 3/Subsystem ==
  G : Inport
  TESUB6 XMNSEA : Subsystem
  TESUB6 XMNSEB : Subsystem
  TESUB6 XMNSEC : Subsystem
  TESUB6 XMNSED : Subsystem
  TESUB6 XMNSEE : Subsystem
  TESUB6 XMNSEF : Subsystem
  TESUB6 XMNSEG : Subsystem
  TESUB6 XMNSEH : Subsystem
  XMNSEA : Outport  VectorParamsAs1DForOutWhenUnconnected=off
  XMNSEB : Outport  Port=2  VectorParamsAs1DForOutWhenUnconnected=off
  XMNSEC : Outport  Port=3  VectorParamsAs1DForOutWhenUnconnected=off
  XMNSED : Outport  Port=4  VectorParamsAs1DForOutWhenUnconnected=off
  XMNSEE : Outport  Port=5  VectorParamsAs1DForOutWhenUnconnected=off
  XMNSEF : Outport  Port=6  VectorParamsAs1DForOutWhenUnconnected=off
  XMNSEG : Outport  Port=7  VectorParamsAs1DForOutWhenUnconnected=off
  XMNSEH : Outport  Port=8  VectorParamsAs1DForOutWhenUnconnected=off
  G_NEW : Outport  Port=9  VectorParamsAs1DForOutWhenUnconnected=off
  wires:
  TESUB6 XMNSEB/2(G_NEW) -> TESUB6 XMNSEC/1(G)
  G/1 -> TESUB6 XMNSEA/1(G)
  TESUB6 XMNSEA/2(G_NEW) -> TESUB6 XMNSEB/1(G)
  TESUB6 XMNSEC/2(G_NEW) -> TESUB6 XMNSED/1(G)
  TESUB6 XMNSED/1(XMNSED) -> XMNSED/1  "XMNSED"
  TESUB6 XMNSEE/1(XMNSEE) -> XMNSEE/1  "XMNSEE"
  TESUB6 XMNSED/2(G_NEW) -> TESUB6 XMNSEE/1(G)
  TESUB6 XMNSEC/1(XMNSEC) -> XMNSEC/1  "XMNSEC"
  TESUB6 XMNSEA/1(XMNSEA) -> XMNSEA/1  "XMNSEA"
  TESUB6 XMNSEB/1(XMNSEB) -> XMNSEB/1  "XMNSEB"
  TESUB6 XMNSEE/2(G_NEW) -> TESUB6 XMNSEF/1(G)
  TESUB6 XMNSEF/2(G_NEW) -> TESUB6 XMNSEG/1(G)
  TESUB6 XMNSEG/2(G_NEW) -> TESUB6 XMNSEH/1(G)
  TESUB6 XMNSEH/2(G_NEW) -> G_NEW/1
  TESUB6 XMNSEF/1(XMNSEF) -> XMNSEF/1  "XMNSEF"
  TESUB6 XMNSEG/1(XMNSEG) -> XMNSEG/1  "XMNSEG"
  TESUB6 XMNSEH/1(XMNSEH) -> XMNSEH/1  "XMNSEH"

== system TEP_Final_NoScript/Random number generator1/Stream Measurements SMEAS Gas analysis/If Action Subsystem3/Subsystem/Stream 4/Subsystem ==
  G : Inport
  TESUB6 XMNSEA : Subsystem
  TESUB6 XMNSEB : Subsystem
  TESUB6 XMNSEC : Subsystem
  TESUB6 XMNSED : Subsystem
  TESUB6 XMNSEE : Subsystem
  TESUB6 XMNSEF : Subsystem
  TESUB6 XMNSEG : Subsystem
  TESUB6 XMNSEH : Subsystem
  XMNSEA : Outport  VectorParamsAs1DForOutWhenUnconnected=off
  XMNSEB : Outport  Port=2  VectorParamsAs1DForOutWhenUnconnected=off
  XMNSEC : Outport  Port=3  VectorParamsAs1DForOutWhenUnconnected=off
  XMNSED : Outport  Port=4  VectorParamsAs1DForOutWhenUnconnected=off
  XMNSEE : Outport  Port=5  VectorParamsAs1DForOutWhenUnconnected=off
  XMNSEF : Outport  Port=6  VectorParamsAs1DForOutWhenUnconnected=off
  XMNSEG : Outport  Port=7  VectorParamsAs1DForOutWhenUnconnected=off
  XMNSEH : Outport  Port=8  VectorParamsAs1DForOutWhenUnconnected=off
  G_NEW : Outport  Port=9  VectorParamsAs1DForOutWhenUnconnected=off
  wires:
  TESUB6 XMNSEB/2(G_NEW) -> TESUB6 XMNSEC/1(G)
  G/1 -> TESUB6 XMNSEA/1(G)
  TESUB6 XMNSEA/2(G_NEW) -> TESUB6 XMNSEB/1(G)
  TESUB6 XMNSEC/2(G_NEW) -> TESUB6 XMNSED/1(G)
  TESUB6 XMNSED/1(XMNSED) -> XMNSED/1  "XMNSED"
  TESUB6 XMNSEE/1(XMNSEE) -> XMNSEE/1  "XMNSEE"
  TESUB6 XMNSED/2(G_NEW) -> TESUB6 XMNSEE/1(G)
  TESUB6 XMNSEC/1(XMNSEC) -> XMNSEC/1  "XMNSEC"
  TESUB6 XMNSEA/1(XMNSEA) -> XMNSEA/1  "XMNSEA"
  TESUB6 XMNSEB/1(XMNSEB) -> XMNSEB/1  "XMNSEB"
  TESUB6 XMNSEE/2(G_NEW) -> TESUB6 XMNSEF/1(G)
  TESUB6 XMNSEF/2(G_NEW) -> TESUB6 XMNSEG/1(G)
  TESUB6 XMNSEG/2(G_NEW) -> TESUB6 XMNSEH/1(G)
  TESUB6 XMNSEH/2(G_NEW) -> G_NEW/1
  TESUB6 XMNSEF/1(XMNSEF) -> XMNSEF/1  "XMNSEF"
  TESUB6 XMNSEG/1(XMNSEG) -> XMNSEG/1  "XMNSEG"
  TESUB6 XMNSEH/1(XMNSEH) -> XMNSEH/1  "XMNSEH"

== system TEP_Final_NoScript/Random number generator1/Stream Measurements SMEAS Gas analysis/If Action Subsystem3/Subsystem/Stream 5/Subsystem ==
  G : Inport
  TESUB6 XMNSEA : Subsystem
  TESUB6 XMNSEB : Subsystem
  TESUB6 XMNSEC : Subsystem
  TESUB6 XMNSED : Subsystem
  TESUB6 XMNSEE : Subsystem
  TESUB6 XMNSEF : Subsystem
  TESUB6 XMNSEG : Subsystem
  TESUB6 XMNSEH : Subsystem
  XMNSEA : Outport  VectorParamsAs1DForOutWhenUnconnected=off
  XMNSEB : Outport  Port=2  VectorParamsAs1DForOutWhenUnconnected=off
  XMNSEC : Outport  Port=3  VectorParamsAs1DForOutWhenUnconnected=off
  XMNSED : Outport  Port=4  VectorParamsAs1DForOutWhenUnconnected=off
  XMNSEE : Outport  Port=5  VectorParamsAs1DForOutWhenUnconnected=off
  XMNSEF : Outport  Port=6  VectorParamsAs1DForOutWhenUnconnected=off
  XMNSEG : Outport  Port=7  VectorParamsAs1DForOutWhenUnconnected=off
  XMNSEH : Outport  Port=8  VectorParamsAs1DForOutWhenUnconnected=off
  G_NEW : Outport  Port=9  VectorParamsAs1DForOutWhenUnconnected=off
  wires:
  TESUB6 XMNSEB/2(G_NEW) -> TESUB6 XMNSEC/1(G)
  G/1 -> TESUB6 XMNSEA/1(G)
  TESUB6 XMNSEA/2(G_NEW) -> TESUB6 XMNSEB/1(G)
  TESUB6 XMNSEC/2(G_NEW) -> TESUB6 XMNSED/1(G)
  TESUB6 XMNSED/1(XMNSED) -> XMNSED/1  "XMNSED"
  TESUB6 XMNSEE/1(XMNSEE) -> XMNSEE/1  "XMNSEE"
  TESUB6 XMNSED/2(G_NEW) -> TESUB6 XMNSEE/1(G)
  TESUB6 XMNSEC/1(XMNSEC) -> XMNSEC/1  "XMNSEC"
  TESUB6 XMNSEA/1(XMNSEA) -> XMNSEA/1  "XMNSEA"
  TESUB6 XMNSEB/1(XMNSEB) -> XMNSEB/1  "XMNSEB"
  TESUB6 XMNSEE/2(G_NEW) -> TESUB6 XMNSEF/1(G)
  TESUB6 XMNSEF/2(G_NEW) -> TESUB6 XMNSEG/1(G)
  TESUB6 XMNSEG/2(G_NEW) -> TESUB6 XMNSEH/1(G)
  TESUB6 XMNSEH/2(G_NEW) -> G_NEW/1
  TESUB6 XMNSEF/1(XMNSEF) -> XMNSEF/1  "XMNSEF"
  TESUB6 XMNSEG/1(XMNSEG) -> XMNSEG/1  "XMNSEG"
  TESUB6 XMNSEH/1(XMNSEH) -> XMNSEH/1  "XMNSEH"

== system TEP_Final_NoScript/Random number generator1/Stream Measurements SMEAS Gas analysis/If Action Subsystem3/Subsystem/Stream 6/Subsystem ==
  G : Inport
  TESUB6 XMNSEA : Subsystem
  TESUB6 XMNSEB : Subsystem
  TESUB6 XMNSEC : Subsystem
  TESUB6 XMNSED : Subsystem
  TESUB6 XMNSEE : Subsystem
  TESUB6 XMNSEF : Subsystem
  TESUB6 XMNSEG : Subsystem
  TESUB6 XMNSEH : Subsystem
  XMNSEA : Outport  VectorParamsAs1DForOutWhenUnconnected=off
  XMNSEB : Outport  Port=2  VectorParamsAs1DForOutWhenUnconnected=off
  XMNSEC : Outport  Port=3  VectorParamsAs1DForOutWhenUnconnected=off
  XMNSED : Outport  Port=4  VectorParamsAs1DForOutWhenUnconnected=off
  XMNSEE : Outport  Port=5  VectorParamsAs1DForOutWhenUnconnected=off
  XMNSEF : Outport  Port=6  VectorParamsAs1DForOutWhenUnconnected=off
  XMNSEG : Outport  Port=7  VectorParamsAs1DForOutWhenUnconnected=off
  XMNSEH : Outport  Port=8  VectorParamsAs1DForOutWhenUnconnected=off
  G_NEW : Outport  Port=9  VectorParamsAs1DForOutWhenUnconnected=off
  wires:
  TESUB6 XMNSEB/2(G_NEW) -> TESUB6 XMNSEC/1(G)
  G/1 -> TESUB6 XMNSEA/1(G)
  TESUB6 XMNSEA/2(G_NEW) -> TESUB6 XMNSEB/1(G)
  TESUB6 XMNSEC/2(G_NEW) -> TESUB6 XMNSED/1(G)
  TESUB6 XMNSED/1(XMNSED) -> XMNSED/1  "XMNSED"
  TESUB6 XMNSEE/1(XMNSEE) -> XMNSEE/1  "XMNSEE"
  TESUB6 XMNSED/2(G_NEW) -> TESUB6 XMNSEE/1(G)
  TESUB6 XMNSEC/1(XMNSEC) -> XMNSEC/1  "XMNSEC"
  TESUB6 XMNSEA/1(XMNSEA) -> XMNSEA/1  "XMNSEA"
  TESUB6 XMNSEB/1(XMNSEB) -> XMNSEB/1  "XMNSEB"
  TESUB6 XMNSEE/2(G_NEW) -> TESUB6 XMNSEF/1(G)
  TESUB6 XMNSEF/2(G_NEW) -> TESUB6 XMNSEG/1(G)
  TESUB6 XMNSEG/2(G_NEW) -> TESUB6 XMNSEH/1(G)
  TESUB6 XMNSEH/2(G_NEW) -> G_NEW/1
  TESUB6 XMNSEF/1(XMNSEF) -> XMNSEF/1  "XMNSEF"
  TESUB6 XMNSEG/1(XMNSEG) -> XMNSEG/1  "XMNSEG"
  TESUB6 XMNSEH/1(XMNSEH) -> XMNSEH/1  "XMNSEH"

== system TEP_Final_NoScript/Random number generator1/Stream Measurements SMEAS Gas analysis/If Action Subsystem3/Subsystem/Stream 8/Subsystem ==
  G : Inport
  TESUB6 XMNSEA : Subsystem
  TESUB6 XMNSEB : Subsystem
  TESUB6 XMNSEC : Subsystem
  TESUB6 XMNSED : Subsystem
  TESUB6 XMNSEE : Subsystem
  TESUB6 XMNSEF : Subsystem
  TESUB6 XMNSEG : Subsystem
  TESUB6 XMNSEH : Subsystem
  XMNSEA : Outport  VectorParamsAs1DForOutWhenUnconnected=off
  XMNSEB : Outport  Port=2  VectorParamsAs1DForOutWhenUnconnected=off
  XMNSEC : Outport  Port=3  VectorParamsAs1DForOutWhenUnconnected=off
  XMNSED : Outport  Port=4  VectorParamsAs1DForOutWhenUnconnected=off
  XMNSEE : Outport  Port=5  VectorParamsAs1DForOutWhenUnconnected=off
  XMNSEF : Outport  Port=6  VectorParamsAs1DForOutWhenUnconnected=off
  XMNSEG : Outport  Port=7  VectorParamsAs1DForOutWhenUnconnected=off
  XMNSEH : Outport  Port=8  VectorParamsAs1DForOutWhenUnconnected=off
  G_NEW : Outport  Port=9  VectorParamsAs1DForOutWhenUnconnected=off
  wires:
  TESUB6 XMNSEB/2(G_NEW) -> TESUB6 XMNSEC/1(G)
  G/1 -> TESUB6 XMNSEA/1(G)
  TESUB6 XMNSEA/2(G_NEW) -> TESUB6 XMNSEB/1(G)
  TESUB6 XMNSEC/2(G_NEW) -> TESUB6 XMNSED/1(G)
  TESUB6 XMNSED/1(XMNSED) -> XMNSED/1  "XMNSED"
  TESUB6 XMNSEE/1(XMNSEE) -> XMNSEE/1  "XMNSEE"
  TESUB6 XMNSED/2(G_NEW) -> TESUB6 XMNSEE/1(G)
  TESUB6 XMNSEC/1(XMNSEC) -> XMNSEC/1  "XMNSEC"
  TESUB6 XMNSEA/1(XMNSEA) -> XMNSEA/1  "XMNSEA"
  TESUB6 XMNSEB/1(XMNSEB) -> XMNSEB/1  "XMNSEB"
  TESUB6 XMNSEE/2(G_NEW) -> TESUB6 XMNSEF/1(G)
  TESUB6 XMNSEF/2(G_NEW) -> TESUB6 XMNSEG/1(G)
  TESUB6 XMNSEG/2(G_NEW) -> TESUB6 XMNSEH/1(G)
  TESUB6 XMNSEH/2(G_NEW) -> G_NEW/1
  TESUB6 XMNSEF/1(XMNSEF) -> XMNSEF/1  "XMNSEF"
  TESUB6 XMNSEG/1(XMNSEG) -> XMNSEG/1  "XMNSEG"
  TESUB6 XMNSEH/1(XMNSEH) -> XMNSEH/1  "XMNSEH"

== system TEP_Final_NoScript/Random number generator1/Stream Measurements SMEAS Gas analysis/If Action Subsystem3/Subsystem/Stream 9/Subsystem ==
  G : Inport
  TESUB6 XMNSEA : Subsystem
  TESUB6 XMNSEB : Subsystem
  TESUB6 XMNSEC : Subsystem
  TESUB6 XMNSED : Subsystem
  TESUB6 XMNSEE : Subsystem
  TESUB6 XMNSEF : Subsystem
  TESUB6 XMNSEG : Subsystem
  TESUB6 XMNSEH : Subsystem
  XMNSEA : Outport  VectorParamsAs1DForOutWhenUnconnected=off
  XMNSEB : Outport  Port=2  VectorParamsAs1DForOutWhenUnconnected=off
  XMNSEC : Outport  Port=3  VectorParamsAs1DForOutWhenUnconnected=off
  XMNSED : Outport  Port=4  VectorParamsAs1DForOutWhenUnconnected=off
  XMNSEE : Outport  Port=5  VectorParamsAs1DForOutWhenUnconnected=off
  XMNSEF : Outport  Port=6  VectorParamsAs1DForOutWhenUnconnected=off
  XMNSEG : Outport  Port=7  VectorParamsAs1DForOutWhenUnconnected=off
  XMNSEH : Outport  Port=8  VectorParamsAs1DForOutWhenUnconnected=off
  G_NEW : Outport  Port=9  VectorParamsAs1DForOutWhenUnconnected=off
  wires:
  TESUB6 XMNSEB/2(G_NEW) -> TESUB6 XMNSEC/1(G)
  G/1 -> TESUB6 XMNSEA/1(G)
  TESUB6 XMNSEA/2(G_NEW) -> TESUB6 XMNSEB/1(G)
  TESUB6 XMNSEC/2(G_NEW) -> TESUB6 XMNSED/1(G)
  TESUB6 XMNSED/1(XMNSED) -> XMNSED/1  "XMNSED"
  TESUB6 XMNSEE/1(XMNSEE) -> XMNSEE/1  "XMNSEE"
  TESUB6 XMNSED/2(G_NEW) -> TESUB6 XMNSEE/1(G)
  TESUB6 XMNSEC/1(XMNSEC) -> XMNSEC/1  "XMNSEC"
  TESUB6 XMNSEA/1(XMNSEA) -> XMNSEA/1  "XMNSEA"
  TESUB6 XMNSEB/1(XMNSEB) -> XMNSEB/1  "XMNSEB"
  TESUB6 XMNSEE/2(G_NEW) -> TESUB6 XMNSEF/1(G)
  TESUB6 XMNSEF/2(G_NEW) -> TESUB6 XMNSEG/1(G)
  TESUB6 XMNSEG/2(G_NEW) -> TESUB6 XMNSEH/1(G)
  TESUB6 XMNSEH/2(G_NEW) -> G_NEW/1
  TESUB6 XMNSEF/1(XMNSEF) -> XMNSEF/1  "XMNSEF"
  TESUB6 XMNSEG/1(XMNSEG) -> XMNSEG/1  "XMNSEG"
  TESUB6 XMNSEH/1(XMNSEH) -> XMNSEH/1  "XMNSEH"

== system TEP_Final_NoScript/Random number generator1/Stream Measurements SMEAS Product analysis/If Action Subsystem3/Subsystem/Subsystem1/Subsystem ==
  G : Inport
  TESUB6 XMNSED : Subsystem
  TESUB6 XMNSEE : Subsystem
  TESUB6 XMNSEF : Subsystem
  TESUB6 XMNSEG : Subsystem
  TESUB6 XMNSEH : Subsystem
  XMNSED : Outport  VectorParamsAs1DForOutWhenUnconnected=off
  XMNSEE : Outport  Port=2  VectorParamsAs1DForOutWhenUnconnected=off
  XMNSEF : Outport  Port=3  VectorParamsAs1DForOutWhenUnconnected=off
  XMNSEG : Outport  Port=4  VectorParamsAs1DForOutWhenUnconnected=off
  XMNSEH : Outport  Port=5  VectorParamsAs1DForOutWhenUnconnected=off
  G_NEW : Outport  Port=6  VectorParamsAs1DForOutWhenUnconnected=off
  wires:
  TESUB6 XMNSEE/2(G_NEW) -> TESUB6 XMNSEF/1(G)
  G/1 -> TESUB6 XMNSED/1(G)
  TESUB6 XMNSED/2(G_NEW) -> TESUB6 XMNSEE/1(G)
  TESUB6 XMNSEF/2(G_NEW) -> TESUB6 XMNSEG/1(G)
  TESUB6 XMNSEG/1(XMNS) -> XMNSEG/1  "XMNSEG"
  TESUB6 XMNSEH/1(XMNS) -> XMNSEH/1  "XMNSEH"
  TESUB6 XMNSEH/2(G_NEW) -> G_NEW/1
  TESUB6 XMNSEG/2(G_NEW) -> TESUB6 XMNSEH/1(G)
  TESUB6 XMNSEF/1(XMNS) -> XMNSEF/1  "XMNSEF"
  TESUB6 XMNSED/1(XMNS) -> XMNSED/1  "XMNSED"
  TESUB6 XMNSEE/1(XMNS) -> XMNSEE/1  "XMNSEE"

== system TEP_Final_NoScript/Random number generator1/Stream Measurements SMEAS Product analysis/If Action Subsystem3/Subsystem/Subsystem2/Subsystem ==
  G : Inport
  TESUB6 XMNSED : Subsystem
  TESUB6 XMNSEE : Subsystem
  TESUB6 XMNSEF : Subsystem
  TESUB6 XMNSEG : Subsystem
  TESUB6 XMNSEH : Subsystem
  XMNSED : Outport  VectorParamsAs1DForOutWhenUnconnected=off
  XMNSEE : Outport  Port=2  VectorParamsAs1DForOutWhenUnconnected=off
  XMNSEF : Outport  Port=3  VectorParamsAs1DForOutWhenUnconnected=off
  XMNSEG : Outport  Port=4  VectorParamsAs1DForOutWhenUnconnected=off
  XMNSEH : Outport  Port=5  VectorParamsAs1DForOutWhenUnconnected=off
  G_NEW : Outport  Port=6  VectorParamsAs1DForOutWhenUnconnected=off
  wires:
  TESUB6 XMNSEE/2(G_NEW) -> TESUB6 XMNSEF/1(G)
  G/1 -> TESUB6 XMNSED/1(G)
  TESUB6 XMNSED/2(G_NEW) -> TESUB6 XMNSEE/1(G)
  TESUB6 XMNSEF/2(G_NEW) -> TESUB6 XMNSEG/1(G)
  TESUB6 XMNSEG/1(XMNS) -> XMNSEG/1  "XMNSEG"
  TESUB6 XMNSEH/1(XMNS) -> XMNSEH/1  "XMNSEH"
  TESUB6 XMNSEH/2(G_NEW) -> G_NEW/1
  TESUB6 XMNSEG/2(G_NEW) -> TESUB6 XMNSEH/1(G)
  TESUB6 XMNSEF/1(XMNS) -> XMNSEF/1  "XMNSEF"
  TESUB6 XMNSED/1(XMNS) -> XMNSED/1  "XMNSED"
  TESUB6 XMNSEE/1(XMNS) -> XMNSEE/1  "XMNSEE"

== system TEP_Final_NoScript/Subsystem/Braatz/ 10/CONTROL 6/P Control/  ==
  DXMV : Inport
  XMV_0 : Inport  Port=2
  XMEAS : Inport  Port=3
  Add : Sum
  Delay : Delay  DelayLength=1  InitialConditionSource=Input port  InitialCondition=0
      settings: InputPortMap=u0,p4
  Pressure limits : Subsystem
      mask Display: color('Blue'),disp('Pressure limits'),
  XMV : Outport
  wires:
  XMV_0/1 -> Delay/2
  Delay/1 -> Add/1
  Add/1 -> Pressure limits/1("XMV(6) ")
  Pressure limits/1(XMV(6)) -> Delay/1, XMV/1
  DXMV/1 -> Add/2
  XMEAS/1 -> Pressure limits/2(XMEAS)

== system TEP_Final_NoScript/Subsystem/Braatz/ 10/CONTROL 6/P Control/ERR ==
  SETPT : Inport
  High Limit : Inport  Port=2
  XMEAS : Inport  Port=3
  " " : Product  Inputs=**/
  Bus Selector : BusSelector  OutputSignals=signal3.XMEAS(10)
  Constant : Constant  Value=100
  Subtract : Sum  Inputs=+-
  ERR : Outport  VectorParamsAs1DForOutWhenUnconnected=off
  wires:
  " "/1 -> ERR/1
  SETPT/1 -> Subtract/1
  Subtract/1 -> " "/1
  High Limit/1 -> " "/3
  Constant/1 -> " "/2
  XMEAS/1 -> Bus Selector/1
  Bus Selector/1 -> Subtract/2  "<XMEAS(10)>"

== system TEP_Final_NoScript/Subsystem/Braatz/ 10/CONTROL 6/P Control/Subsystem ==
  ERR : Inport
  GAIN : Inport  Port=2
  ERROLD : UnitDelay  SampleTime=-1  HasFrameUpgradeWarning=on
  Product : Product
  Subtract1 : Sum  Inputs=+-
  DXMV : Outport  VectorParamsAs1DForOutWhenUnconnected=off
  wires:
  ERR/1 -> Subtract1/1, ERROLD/1
  ERROLD/1 -> Subtract1/2
  Subtract1/1 -> Product/2
  Product/1 -> DXMV/1
  GAIN/1 -> Product/1

== system TEP_Final_NoScript/Random number generator1/Stream Measurements SMEAS Gas analysis/If Action Subsystem3/Subsystem/Stream 1/Subsystem/TESUB6 XMNSEA ==
  G : Inport
  Process Noise I=1-12 G New : mylib/Process Noise I=1-12 G New  SystemSampleTime=-1  VariantActivationTime=update diagram  AllowFlexibleInterface=on  Latency=0  AutoFrameSizeCalculation=off
      settings: SourceProductName=TEP Library
  XNSEA : Constant  Value=0.25
  XMNSEA : Outport  VectorParamsAs1DForOutWhenUnconnected=off
  G_NEW : Outport  Port=2  VectorParamsAs1DForOutWhenUnconnected=off
  wires:
  XNSEA/1 -> Process Noise I=1-12 G New/1
  Process Noise I=1-12 G New/1 -> XMNSEA/1
  G/1 -> Process Noise I=1-12 G New/2
  Process Noise I=1-12 G New/2 -> G_NEW/1

== system TEP_Final_NoScript/Random number generator1/Stream Measurements SMEAS Gas analysis/If Action Subsystem3/Subsystem/Stream 1/Subsystem/TESUB6 XMNSEB ==
  G : Inport
  Process Noise I=1-12 G New : mylib/Process Noise I=1-12 G New  SystemSampleTime=-1  VariantActivationTime=update diagram  AllowFlexibleInterface=on  Latency=0  AutoFrameSizeCalculation=off
      settings: SourceProductName=TEP Library
  XNSEB : Constant  Value=0.1
  XMNSEB : Outport  VectorParamsAs1DForOutWhenUnconnected=off
  G_NEW : Outport  Port=2  VectorParamsAs1DForOutWhenUnconnected=off
  wires:
  XNSEB/1 -> Process Noise I=1-12 G New/1
  Process Noise I=1-12 G New/1 -> XMNSEB/1
  G/1 -> Process Noise I=1-12 G New/2
  Process Noise I=1-12 G New/2 -> G_NEW/1
